simulink model "Dubinscar"  (R2023b)
settings: Solver=VariableStepAuto  StartTime=0.0  StopTime=10.0  RelTol=1e-3
settings Model: Creator=24246  LastModifiedBy=24246

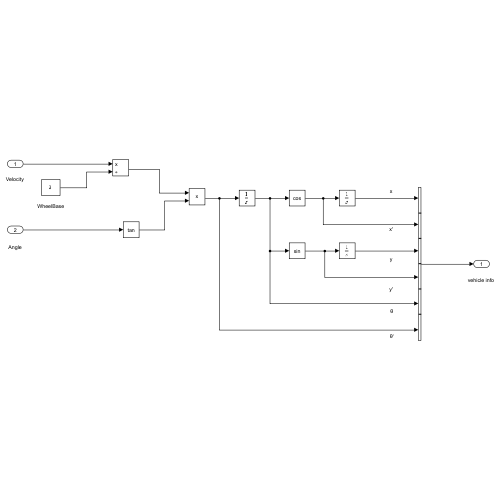
[thumbnail: Simulink's stored preview of the top-level diagram]
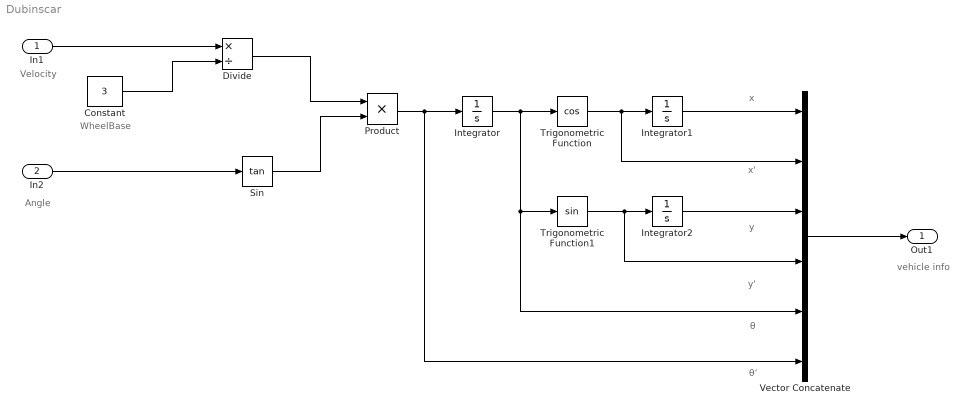
== system Dubinscar ==
  note: vehicle info
  note: θ‘
  note: θ
  note: y'
  note: y
  note: x'
  note: x
  note: WheelBase
  note: Angle
  note: Velocity
  In1 : Inport
  In2 : Inport  Port=2
  Constant : Constant  Value=3
  Divide : Product  Inputs=*/
  Integrator : Integrator
  Integrator1 : Integrator
  Integrator2 : Integrator
  Product : Product
  Sin : Trigonometry  Operator=tan
  Trigonometric Function : Trigonometry  Operator=cos
  Trigonometric Function1 : Trigonometry
  Vector Concatenate : Concatenate  NumInputs=6
  Out1 : Outport
  wires:
  In1/1 -> Divide/1
  Constant/1 -> Divide/2
  In2/1 -> Sin/1
  Divide/1 -> Product/1
  Sin/1 -> Product/2
  Product/1 -> Vector Concatenate/6, Integrator/1
  Integrator/1 -> Vector Concatenate/5, Trigonometric Function1/1, Trigonometric Function/1
  Trigonometric Function/1 -> Vector Concatenate/2, Integrator1/1
  Integrator1/1 -> Vector Concatenate/1
  Trigonometric Function1/1 -> Vector Concatenate/4, Integrator2/1
  Integrator2/1 -> Vector Concatenate/3
  Vector Concatenate/1 -> Out1/1
